simulink model "automodell"  (R2016b)
settings: Solver=VariableStepAuto  StartTime=0.0  StopTime=150  RelTol=1e-3
values from neighbouring files (symbols this model uses):
  C = 0.6    [automodell_param.m]    (also in serienschwingkreis_param.m = 0.005)
  Fan = 3000    [automodell_param.m]
  Froll = 250    [automodell_param.m]
  m = 1500    [automodell_param.m]
settings Model: Creator=local  LastModifiedBy=local

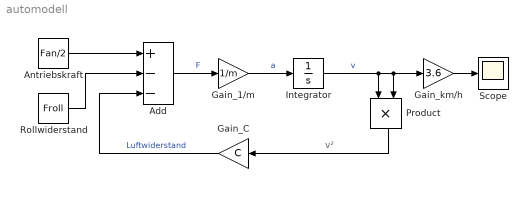
== system automodell ==
  note: v²
  Add : Sum  Inputs=+--
  Antriebskraft : Constant  Value=Fan/2
  Gain_1/m : Gain  Gain=1/m
  Gain_C : Gain  Gain=C
  Gain_km/h : Gain  Gain=3.6
  Integrator : Integrator
  Product : Product
  Rollwiderstand : Constant  Value=Froll
  Scope : Scope
  wires:
  Antriebskraft/1 -> Add/1
  Add/1 -> Gain_1/m/1  "F"
  Rollwiderstand/1 -> Add/2
  Gain_1/m/1 -> Integrator/1  "a"
  Integrator/1 -> Gain_km/h/1, Product/2, Product/1  "v"
  Product/1 -> Gain_C/1
  Gain_C/1 -> Add/3  "Luftwiderstand"
  Gain_km/h/1 -> Scope/1
